simulink model "actgr"  (R2024a)
settings: Solver=ode45  StartTime=0.0  StopTime=8  MaxStep=1e-3  RelTol=1e-5
model workspace (MAT data in the model file):
  E0 = 10
  EC50 = 9.98
  Emax = 5.17
  F = 0.89
  K = 0.28
  K12 = 1.78
  K21 = 2.2
  Ka = 1.8
  Ke0 = 0.83
  Ke1 = 0.83
settings Model: Creator=pablo  LastModifiedBy=pablo

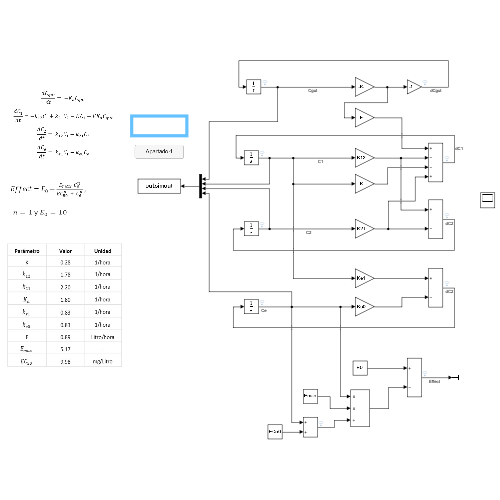
[thumbnail: Simulink's stored preview of the top-level diagram]
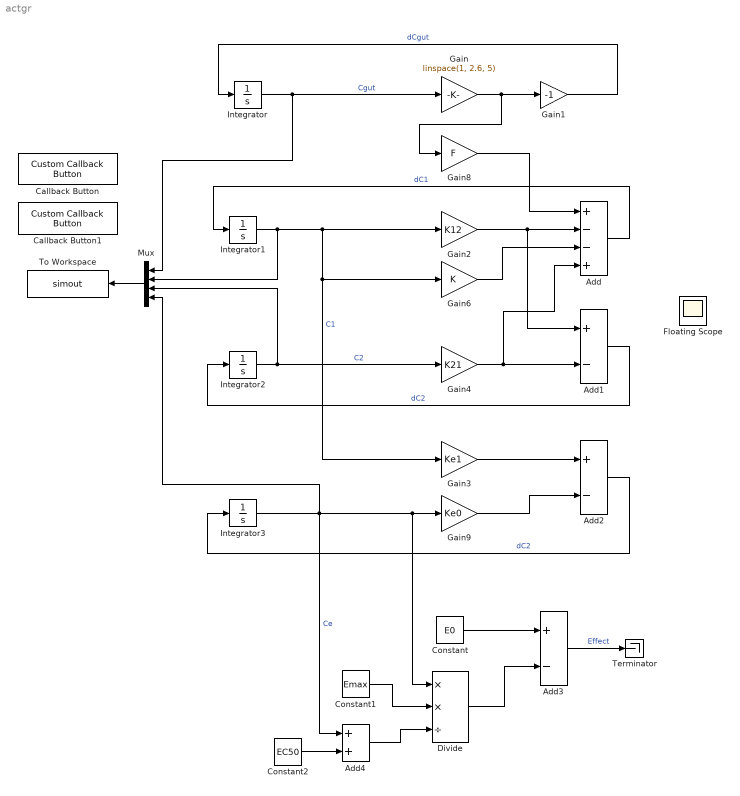
== system actgr ==
  Add : Sum  Inputs=+--+
  Add1 : Sum  Inputs=+-
  Add2 : Sum  Inputs=+-
  Add3 : Sum  Inputs=+-
  Add4 : Sum
  Callback Button : CustomCallbackButton  Configuration="{\"components\":[{\"name\":\"BackgroundImageComponent\",\"settings\":{\"image\":{\"size\":[0,0],\"src\":\"default\",\"srcOrientation\":\"Right\"},\"position\":[0,0,1,1]}},{\"name\":\"ButtonStateComponent\",\"settings\":{\"buttonType\":\"momentary\",\"clickFcn\":\"close all;\\n\\nwholesize = size(out.simout);\\ntsize = wholesize(1);\\nnvar = wholesize(2)\\/4; \\nt = 1\\/1000:1\\/1000:tsize\\/1000;\\nt = t';\\n\\nCgut = zeros(tsize, nvar);\\nC1 = zeros(tsize, nvar);\\nC2 = zeros(tsize, nvar);\\nCe = zeros(tsize, nvar);\\nEffect = zeros(tsize, nvar);\\n\\nE0 = 10;\\nEmax = 5.17;\\nEC50 = 9.98;\\n\\n\\nfor i=1:nvar\\n    Cgut(:, i) = out.simout(:, i+0*nvar);\\n    C1(:, i) = out.simout(:, i+1*nvar);\\n    C2(:, i) = out.simout(:,i+2*nvar);\\n    Ce(:, i) = out.simout(:,i+3*nvar);\\n\\n    Effect(:, i) = E0 - ((Emax*Ce(:, i)).\\/(EC50 + Ce(:, i)));\\nend\\n\\n[Cgutmax, iCgutmax] = max(Cgut);\\n[C1max, iC1max] = max(C1);\\n[C2max, iC2max] = max(C2);\\n[Cemax, iCemax]  = max(Ce);\\n[Effectmax, iEffectmax]  = min(Effect);\\n\\nfigure(1)\\nplot(t, C1, 'b')\\nhold on\\nplot(t, Ce, 'r')\\nplot(iC1max\\/1000, C1max, 'b*', 'MarkerSize', 10, 'MarkerFaceColor', 'r'); \\nplot(iCemax\\/1000, Cemax, 'r*', 'MarkerSize', 10, 'MarkerFaceColor', 'r'); \\ngrid on\\n\\nfigure(2)\\nplot(t, Effect, 'g')\\nhold on\\nplot(iEffectmax\\/1000, Effectmax, 'g*', 'MarkerSize', 10, 'MarkerFaceColor', 'r');\\ngrid on\",\"onValue\":1,\"position\":[0,0,1,1],\"pressDelay\":\"500\",\"pressFcn\":\"\",\"repeatInterval\":\"0\",\"states\":[{\"horizontalAlignment\":\"center\",\"image\":{\"position\":[0,0,1,1],\"size\":[1,1],\"src\":\"default\",\"srcOrientation\":\"Right\"},\"label\":{\"color\":[0.01176470588,0.01176470588,0.01176470588,1],\"icon\":{\"size\":[0,0],\"src\":\"default\",\"srcOrientation\":\"Right\"},\"iconPlacement\":\"left\",\"opacity\":1,\"show\":true,\"text\":{\"content\":\"Apartados 3 y 5\",\"font\":\"Helvetica\",\"fontSize\":15}},\"labelOffset\":[0,0],\"verticalAlignment\":\"middle\"},{\"horizontalAlignment\":\"center\",\"image\":{\"position\":[0,0,1,1],\"size\":[1,1],\"src\":\"default\",\"srcOrientation\":\"Right\"},\"label\":{\"color\":[0.01176470588,0.01176470588,0.01176470588,1],\"icon\":{\"size\":[0,0],\"src\":\"default\",\"srcOrientation\":\"Right\"},\"iconPlacement\":\"left\",\"opacity\":1,\"show\":true,\"text\":{\"content\":\"Apartados 3 y 5\",\"font\":\"Helvetica\",\"fontSize\":15}},\"labelOffset\":[0,0],\"verticalAlignment\":\"middle\"},{\"horizontalAlignment\":\"center\",\"image\":{\"position\":[0,0,1,1],\"size\":[1,1],\"src\":\"default\",\"srcOrientation\":\"Right\"},\"label\":{\"color\":[0.01176470588,0.01176470588,0.01176470588,1],\"icon\":{\"size\":[0,0],\"src\":\"default\",\"srcOrientation\":\"Right\"},\"iconPlacement\":\"left\",\"opacity\":1,\"show\":true,\"text\":{\"content\":\"Apartados 3 y 5\",\"font\":\"Helvetica\",\"fontSize\":15}},\"labelOffset\":[0,0],\"verticalAlignment\":\"middle\"},{\"horizontalAlignment\":\"center\",\"image\":{\"position\":[0,0,1,1],\"size\":[1,1],\"src\":\"default\",\"srcOrientation\":\"Right\"},\"label\":{\"color\":[0.01176470588,0.01176470588,0.01176470588,1],\"icon\":{\"size\":[0,0],\"src\":\"default\",\"srcOrientation\":\"Right\"},\"iconPlacement\":\"left\",\"opacity\":1,\"show\":true,\"text\":{\"content\":\"Apartados 3 y 5\",\"font\":\"Helvetica\",\"fontSize\":15}},\"labelOffset\":[0,0],\"verticalAlignment\":\"middle\"}]}},{\"name\":\"ForegroundImageComponent\",\"settings\":{\"image\":{\"size\":[0,0],\"src\":\"default\",\"srcOrientation\":\"Right\"},\"isForeground\":1,\"position\":[0,0,1,1]}}],\"settings\":{\"BindingType\":\"standalone\",\"backgroundColor\":[244,244,244,1],\"backgroundOffset\":0.2,\"backgroundOpacity\":1,\"fixedAspectRatio\":\"off\",\"foregroundColor\":[0.01176470588,0.01176470588,0.01176470588,1],\"migratedFromLegacy\":true,\"useBackgroundColor\":true,\"variant\":\"callback\",\"version\":\"R2023a\"},\"type\":\"Button\"}"  CustomBackgroundColor="{\"color\":[0.9568627451,0.9568627451,0.9568627451],\"show\":true}"
  Callback Button1 : CustomCallbackButton  Configuration="{\"components\":[{\"name\":\"BackgroundImageComponent\",\"settings\":{\"image\":{\"size\":[0,0],\"src\":\"default\",\"srcOrientation\":\"Right\"},\"position\":[0,0,1,1]}},{\"name\":\"ButtonStateComponent\",\"settings\":{\"buttonType\":\"momentary\",\"clickFcn\":\"close all;\\n\\nwholesize = size(out.simout);\\ntsize = wholesize(1);\\nnvar = 5; \\nt = 1\\/1000:1\\/1000:tsize\\/1000;\\nt = t';\\n\\nCgut = zeros(tsize, 1);\\nC1 = zeros(tsize, nvar);\\nC2 = zeros(tsize, nvar);\\nCe = zeros(tsize, nvar);\\nEffect = zeros(tsize, nvar);\\n\\nE0 = 10;\\nEmax = 5.17;\\nEC50 = 9.98;\\n\\nCgut = out.simout(:, 1);\\n\\nfor i=1:nvar\\n    C1(:, i) = out.simout(:, i+0*nvar+1);\\n    C2(:, i) = out.simout(:,i+1*nvar+1);\\n    Ce(:, i) = out.simout(:,i+2*nvar+1);\\n\\n    Effect(:, i) = E0 - ((Emax*Ce(:, i)).\\/(EC50 + Ce(:, i)));\\nend\\n\\n[Cgutmax, iCgutmax] = max(Cgut);\\n[C1max, iC1max] = max(C1);\\n[C2max, iC2max] = max(C2);\\n[Cemax, iCemax]  = max(Ce);\\n[Effectmax, iEffectmax]  = min(Effect);\\n\\nfigure(1)\\nplot(t, C1, 'b')\\nhold on\\nplot(t, Ce, 'r')\\nplot(iC1max\\/1000, C1max, 'b*', 'MarkerSize', 10, 'MarkerFaceColor', 'r'); \\nplot(iCemax\\/1000, Cemax, 'r*', 'MarkerSize', 10, 'MarkerFaceColor', 'r'); \\ngrid on\\n\\nfigure(2)\\nplot(t, Effect, 'g')\\nhold on\\nplot(iEffectmax\\/1000, Effectmax, 'g*', 'MarkerSize', 10, 'MarkerFaceColor', 'r'); \\ngrid on\",\"onValue\":1,\"position\":[0,0,1,1],\"pressDelay\":\"500\",\"pressFcn\":\"\",\"repeatInterval\":\"0\",\"states\":[{\"horizontalAlignment\":\"center\",\"image\":{\"position\":[0,0,1,1],\"size\":[1,1],\"src\":\"default\",\"srcOrientation\":\"Right\"},\"label\":{\"color\":[0.01176470588,0.01176470588,0.01176470588,1],\"icon\":{\"size\":[0,0],\"src\":\"default\",\"srcOrientation\":\"Right\"},\"iconPlacement\":\"left\",\"opacity\":1,\"show\":true,\"text\":{\"content\":\"Apartado 4\",\"font\":\"Helvetica\",\"fontSize\":15}},\"labelOffset\":[0,0],\"verticalAlignment\":\"middle\"},{\"horizontalAlignment\":\"center\",\"image\":{\"position\":[0,0,1,1],\"size\":[1,1],\"src\":\"default\",\"srcOrientation\":\"Right\"},\"label\":{\"color\":[0.01176470588,0.01176470588,0.01176470588,1],\"icon\":{\"size\":[0,0],\"src\":\"default\",\"srcOrientation\":\"Right\"},\"iconPlacement\":\"left\",\"opacity\":1,\"show\":true,\"text\":{\"content\":\"Apartado 4\",\"font\":\"Helvetica\",\"fontSize\":15}},\"labelOffset\":[0,0],\"verticalAlignment\":\"middle\"},{\"horizontalAlignment\":\"center\",\"image\":{\"position\":[0,0,1,1],\"size\":[1,1],\"src\":\"default\",\"srcOrientation\":\"Right\"},\"label\":{\"color\":[0.01176470588,0.01176470588,0.01176470588,1],\"icon\":{\"size\":[0,0],\"src\":\"default\",\"srcOrientation\":\"Right\"},\"iconPlacement\":\"left\",\"opacity\":1,\"show\":true,\"text\":{\"content\":\"Apartado 4\",\"font\":\"Helvetica\",\"fontSize\":15}},\"labelOffset\":[0,0],\"verticalAlignment\":\"middle\"},{\"horizontalAlignment\":\"center\",\"image\":{\"position\":[0,0,1,1],\"size\":[1,1],\"src\":\"default\",\"srcOrientation\":\"Right\"},\"label\":{\"color\":[0.01176470588,0.01176470588,0.01176470588,1],\"icon\":{\"size\":[0,0],\"src\":\"default\",\"srcOrientation\":\"Right\"},\"iconPlacement\":\"left\",\"opacity\":1,\"show\":true,\"text\":{\"content\":\"Apartado 4\",\"font\":\"Helvetica\",\"fontSize\":15}},\"labelOffset\":[0,0],\"verticalAlignment\":\"middle\"}]}},{\"name\":\"ForegroundImageComponent\",\"settings\":{\"image\":{\"size\":[0,0],\"src\":\"default\",\"srcOrientation\":\"Right\"},\"isForeground\":1,\"position\":[0,0,1,1]}}],\"settings\":{\"BindingType\":\"standalone\",\"backgroundColor\":[244,244,244,1],\"backgroundOffset\":0.2,\"backgroundOpacity\":1,\"fixedAspectRatio\":\"off\",\"foregroundColor\":[0.01176470588,0.01176470588,0.01176470588,1],\"migratedFromLegacy\":true,\"useBackgroundColor\":true,\"variant\":\"callback\",\"version\":\"R2023a\"},\"type\":\"Button\"}"  CustomBackgroundColor="{\"color\":[0.9568627451,0.9568627451,0.9568627451],\"show\":true}"
  Constant : Constant  Value=E0
  Constant1 : Constant  Value=Emax
  Constant2 : Constant  Value=EC50
  Divide : Product  Inputs=**/
  Floating Scope : Scope
      settings: Floating=on
  Gain : Gain  Gain=linspace(1, 2.6, 5)
  Gain1 : Gain  Gain=-1
  Gain2 : Gain  Gain=K12
  Gain3 : Gain  Gain=Ke1
  Gain4 : Gain  Gain=K21
  Gain6 : Gain  Gain=K
  Gain8 : Gain  Gain=F
  Gain9 : Gain  Gain=Ke0
  Integrator : Integrator  InitialCondition=200
  Integrator1 : Integrator
  Integrator2 : Integrator
  Integrator3 : Integrator
  Mux : Mux
  Terminator : Terminator
  To Workspace : ToWorkspace  VariableName=simout  SampleTime=-1
  wires:
  Integrator/1 -> Gain/1, Mux/1  "Cgut"
  Integrator1/1 -> Gain2/1, Gain6/1, Gain3/1, Mux/2  "C1"
  Integrator2/1 -> Gain4/1, Mux/3  "C2"
  Integrator3/1 -> Divide/1, Gain9/1, Mux/4, Add4/1  "Ce"
  Gain/1 -> Gain8/1, Gain1/1
  Gain2/1 -> Add/2, Add1/1
  Gain4/1 -> Add/4, Add1/2
  Gain6/1 -> Add/3
  Gain8/1 -> Add/1
  Add/1 -> Integrator1/1  "dC1"
  Add1/1 -> Integrator2/1  "dC2"
  Gain3/1 -> Add2/1
  Gain9/1 -> Add2/2
  Add2/1 -> Integrator3/1  "dC2"
  Gain1/1 -> Integrator/1  "dCgut"
  Constant1/1 -> Divide/2
  Constant/1 -> Add3/1
  Divide/1 -> Add3/2
  Constant2/1 -> Add4/2
  Add4/1 -> Divide/3
  Add3/1 -> Terminator/1  "Effect"
  Mux/1 -> To Workspace/1
